simulink model "WindMPPTTestHarness"  (R2025a)
settings: Solver=VariableStepAuto  StartTime=0.0  StopTime=15  RelTol=1e-3
model workspace (MAT data in the model file):
  omega = 1500
  windSpeed = 12
libraries: fl_lib x8, nesl_utility x6, simulink x1, ee_lib x1
settings Model: Creator=skota  LastModifiedBy=skota
settings DataIOCC: SaveOutput=off  DSMLogging=off  SaveTime=off  OutputSaveName=windTestHarness

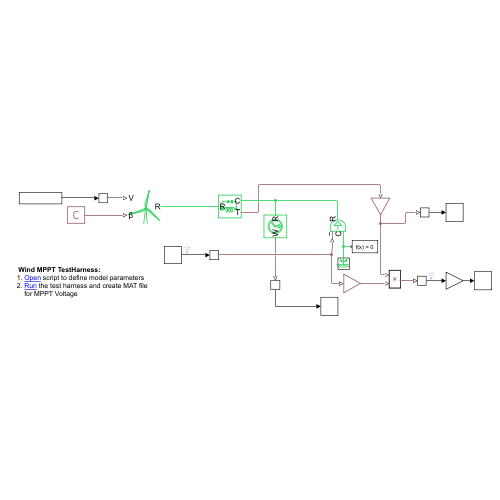
[thumbnail: Simulink's stored preview of the top-level diagram]
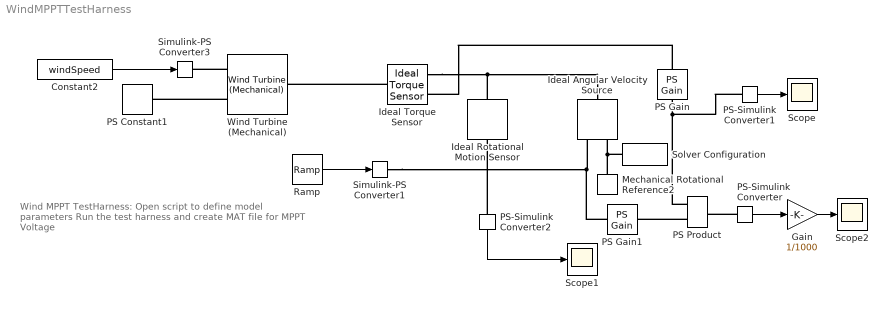
== system WindMPPTTestHarness ==
  note: Wind MPPT TestHarness:
      | Open script to define model parameters
      | Run the test harness and create MAT file for MPPT Voltage
  Constant2 : Constant  Value=windSpeed
  Gain : Gain  Gain=1/1000
  Ideal Angular Velocity Source : fl_lib/Mechanical/Mechanical Sources/Ideal Angular Velocity Source
  Ideal Rotational Motion Sensor : fl_lib/Mechanical/Mechanical Sensors/Ideal Rotational Motion Sensor  reference=foundation.enum.MeasurementReference.absolute  acceleration_port=false  velocity_port=true  position_port=false  wrap_angle=false  offset=0 rad
      settings: InternalSimscapePortConfiguration="{\"Bottom\":[],\"Left\":[{\"id\":\"R\",\"label\":\"R\",\"type\":\"foundation.mechanical.rotational.rotational\"}],\"Right\":[{\"id\":\"W\",\"label\":\"W\",\"type\":\"output\"}],\"Top\":[]}"
  Ideal Torque Sensor : fl_lib/Mechanical/Mechanical Sensors/Ideal Torque Sensor
  Mechanical Rotational Reference2 : fl_lib/Mechanical/Rotational Elements/Mechanical Rotational Reference
  PS Constant1 : fl_lib/Physical Signals/Sources/PS Constant  constant=0
  PS Gain : fl_lib/Physical Signals/Functions/PS Gain  gain=1
  PS Gain1 : fl_lib/Physical Signals/Functions/PS Gain  gain=pi/30
  PS Product : fl_lib/Physical Signals/Functions/PS Product
  PS-Simulink Converter : nesl_utility/PS-Simulink Converter  PhysicalDomain=network_engine_domain  SubClassName=ps_output  LeftPortType=input  RightPortType=output  PseudoPeriodic=off  Frequencies=[]  VectorFormat=inherit  Unit=inherit  AffineConversion=off
  PS-Simulink Converter1 : nesl_utility/PS-Simulink Converter  PhysicalDomain=network_engine_domain  SubClassName=ps_output  LeftPortType=input  RightPortType=output  PseudoPeriodic=off  Frequencies=[]  VectorFormat=inherit  Unit=inherit  AffineConversion=off
  PS-Simulink Converter2 : nesl_utility/PS-Simulink Converter  PhysicalDomain=network_engine_domain  SubClassName=ps_output  LeftPortType=input  RightPortType=output  PseudoPeriodic=off  Frequencies=[]  VectorFormat=inherit  Unit=inherit  AffineConversion=off
  Ramp : simulink/Sources/Ramp  slope=100  start=0  InitialOutput=0
  Scope : Scope
      settings: ActiveDisplayYMinimum=-115.58185  ActiveDisplayYMaximum=1040.23667
  Scope1 : Scope
      settings: ActiveDisplayYMinimum=-19.63495  ActiveDisplayYMaximum=176.71459  DataLoggingVariableName=ScopeData3
  Scope2 : Scope
      settings: ActiveDisplayYMinimum=-6.24829  ActiveDisplayYMaximum=56.23457
  Simulink-PS Converter1 : nesl_utility/Simulink-PS Converter  PhysicalDomain=network_engine_domain  SubClassName=ps_input  LeftPortType=input  RightPortType=output  PseudoPeriodic=off  Frequencies=[]  NoiseDistribution=none  NoiseParameters=[]  Unit=rpm  AffineConversion=off  FilteringAndDerivatives=provide  SimscapeFilterOrder=1  InputFilterTimeConstant=0.001  UdotUserProvided=0
  Simulink-PS Converter3 : nesl_utility/Simulink-PS Converter  PhysicalDomain=network_engine_domain  SubClassName=ps_input  LeftPortType=input  RightPortType=output  PseudoPeriodic=off  Frequencies=[]  NoiseDistribution=none  NoiseParameters=[]  Unit=m/s  AffineConversion=off  FilteringAndDerivatives=provide  SimscapeFilterOrder=1  InputFilterTimeConstant=0.001  UdotUserProvided=0
  Solver Configuration : nesl_utility/Solver Configuration  PhysicalDomain=network_engine_domain  SubClassName=solver  LeftPortType=input  RightPortType=generic  Tones=[]  Harmonics=[]  SimulateNoise=off  Profile=off  UseLocalSampling=off  EnableSwitchedLinearOptims=on  FrequencyDomain=off  UseCCode=off  RelTol=0.001  AbsTol=0.001  MinStep=1e-09  ToWorkspace=off  RevertToSquareIcSolve=off  NumHomotopyIterations=100  PhasorMode=off  PhasorModeNumHarmonics=1  ConsistencySolver=NEWTON_XTOL_AFTER_FTOL  IndexReductionMethod=DerivativeReplacement  DoDC=off  ResidualTolerance=1e-09  ConsistencyTolSource=LOCAL  ConsistencyAbsTol=0.001  ConsistencyRelTol=0.001  ConsistencyTolFactor=0.001  UseLocalSolver=on  LocalSolverChoice=NE_BACKWARD_EULER_ADVANCER  ResolveIndetEquations=on  FunctionEvalNumThread=1  LocalSolverSampleTime=0.001  DoFixedCost=on  MaxNonlinIter=3  MaxModeIter=2  ComputeImpulses=off  ImpulseIterations=2  LinearAlgebra=auto  LinearAlgebraNumThread=0  EquationFormulation=NE_TIME_EF  DelaysMemoryBudget=1024  AutomaticFiltering=on  FilteringTimeConstant=0.001  PartitionStorageMethod=AS_NEEDED  PartitionMemoryBudget=1024  PartitionMethod=ROBUST  MultibodyUseLocalSolver=off  MultibodyLocalSolverChoice=ODE1  MultibodyLocalSolverSampleTime=0.001
  Wind Turbine (Mechanical) : ee_lib/Electromechanical/Wind Turbine (Mechanical)  R_rotor=5.58 m  pitch_TLU=pitch deg  lambda_TLU=tsr  Cp_TLU=cp  v_thr=0.01 m/s  w_thr=0.01 rad/s  rho_air=1.225 kg/m^3  includeInertia=false  J=1 kg*m^2  lam=0 N*m*s/rad  w_specify=off  w_priority=None  w=0 rad/s  w_nominal_specify=off  w_nominal_value=1  w_nominal_unit=rad/s  t_specify=off  t_priority=None  t=0 N*m  t_nominal_specify=off  t_nominal_value=1  t_nominal_unit=N*m  Torque_specify=off  Torque_priority=None  Torque=0 N*m  Torque_nominal_specify=off  Torque_nominal_value=1  Torque_nominal_unit=N*m
      settings: InternalSimscapePortConfiguration="{\"Bottom\":[],\"Left\":[{\"id\":\"vWind\",\"label\":\"V\",\"type\":\"input\"},{\"id\":\"pitch\",\"label\":\"β\",\"type\":\"input\"}],\"Right\":[{\"id\":\"R\",\"label\":\"R\",\"type\":\"foundation.mechanical.rotational.rotational\"}],\"Top\":[]}"
  wires:
  PS-Simulink Converter2/1 -> Scope1/1
  PS-Simulink Converter/1 -> Gain/1
  Gain/1 -> Scope2/1
  Constant2/1 -> Simulink-PS Converter3/1
  Ramp/1 -> Simulink-PS Converter1/1
  PS-Simulink Converter1/1 -> Scope/1
  connections:
  Ideal Rotational Motion Sensor/LConn1 -- Ideal Torque Sensor/RConn1 -- Ideal Angular Velocity Source/LConn1
  PS Product/LConn1 -- PS-Simulink Converter1/LConn1 -- PS Gain/RConn1
  PS-Simulink Converter2/LConn1 -- Ideal Rotational Motion Sensor/RConn1
  PS Gain/LConn1 -- Ideal Torque Sensor/RConn2
  Mechanical Rotational Reference2/LConn1 -- Solver Configuration/RConn1 -- Ideal Angular Velocity Source/RConn2
  Wind Turbine (Mechanical)/LConn2 -- PS Constant1/RConn1
  PS-Simulink Converter/LConn1 -- PS Product/RConn1
  Ideal Torque Sensor/LConn1 -- Wind Turbine (Mechanical)/RConn1
  Wind Turbine (Mechanical)/LConn1 -- Simulink-PS Converter3/RConn1
  PS Product/LConn2 -- PS Gain1/RConn1
  PS Gain1/LConn1 -- Simulink-PS Converter1/RConn1 -- Ideal Angular Velocity Source/RConn1
